simulink model "exploratory_journey"  (R2016a)
settings: Solver=FixedStepAuto  StartTime=0.0  StopTime=Param.T  FixedStep=Param.deltaT  RelTol=1e-3
undefined symbols (not defined in the file or in its folder): drawExpPath, Param, updateExpPosn, X, Y, Z
libraries: robotlib x6
settings Model: Creator=Emily  LastModifiedBy=Emily

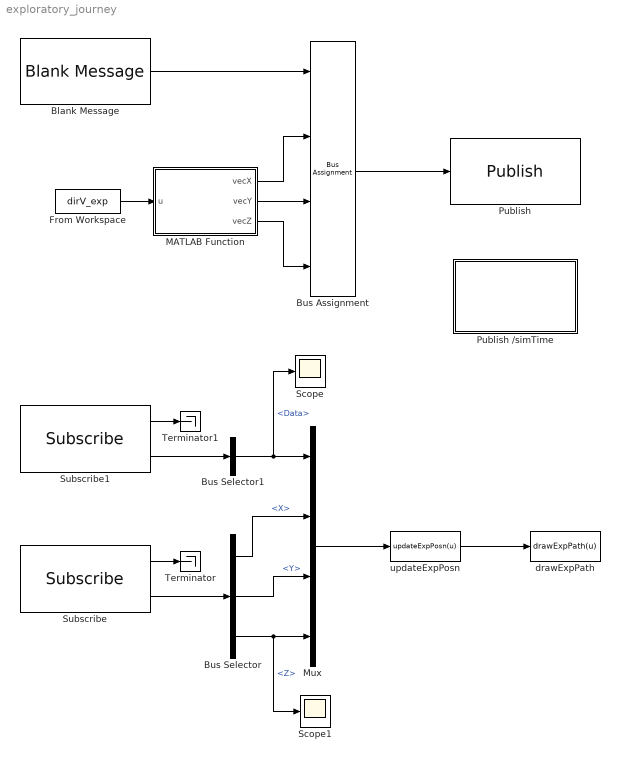
== system exploratory_journey ==
  Blank Message : robotlib/Blank Message  SourceLibraryInfo=This block requires Robotics System Toolbox  messageType=geometry_msgs/Vector3  SampleTime=inf
  Bus Assignment : BusAssignment  AssignedSignals=X,Y,Z
  Bus Selector : BusSelector  OutputSignals=X,Y,Z
  Bus Selector1 : BusSelector  OutputSignals=Data
  From Workspace : FromWorkspace  VariableName=dirV_exp  SampleTime=Param.deltaT  OutputAfterFinalValue=Holding final value
  MATLAB Function : MATLAB Function  TreatAsAtomicUnit=on
  Mux : Mux  Inputs=[1 1 1 1]
  Publish : robotlib/Publish  SourceLibraryInfo=This block requires Robotics System Toolbox  topicSource=Specify your own  topic=/simDir  messageType=geometry_msgs/Vector3  messageQueueLength=1
  Publish /simTime : Subsystem
  Scope : Scope
  Scope1 : Scope
  Subscribe : robotlib/Subscribe  SourceLibraryInfo=This block requires Robotics System Toolbox  topicSource=Specify your own  topic=/simDir  messageType=geometry_msgs/Vector3  sampleTime=-1  messageQueueLength=1
  Subscribe1 : robotlib/Subscribe  SourceLibraryInfo=This block requires Robotics System Toolbox  topicSource=Specify your own  topic=/simTime  messageType=std_msgs/Float64  sampleTime=-1  messageQueueLength=1
  Terminator : Terminator
  Terminator1 : Terminator
  drawExpPath : MATLABFcn  MATLABFcn=drawExpPath(u)  OutputDimensions=0
  updateExpPosn : MATLABFcn  MATLABFcn=updateExpPosn(u)  OutputDimensions=4
  wires:
  Blank Message/1 -> Bus Assignment/1
  Bus Assignment/1 -> Publish/1
  Subscribe/1 -> Terminator/1
  Subscribe/2 -> Bus Selector/1
  Subscribe1/1 -> Terminator1/1
  Subscribe1/2 -> Bus Selector1/1
  Mux/1 -> updateExpPosn/1
  updateExpPosn/1 -> drawExpPath/1
  Bus Selector1/1 -> Scope/1, Mux/1  "<Data>"
  Bus Selector/1 -> Mux/2  "<X>"
  Bus Selector/2 -> Mux/3  "<Y>"
  Bus Selector/3 -> Scope1/1, Mux/4  "<Z>"
  From Workspace/1 -> MATLAB Function/1(u)
  MATLAB Function/2(vecY) -> Bus Assignment/3
  MATLAB Function/1(vecX) -> Bus Assignment/2
  MATLAB Function/3(vecZ) -> Bus Assignment/4

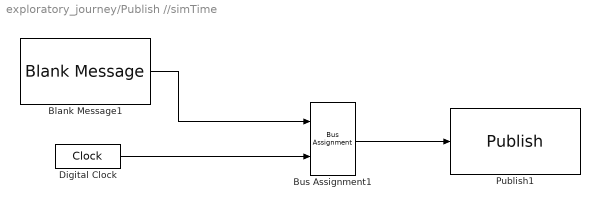
== system exploratory_journey/Publish //simTime ==
  Blank Message1 : robotlib/Blank Message  SourceLibraryInfo=This block requires Robotics System Toolbox  messageType=std_msgs/Float64  SampleTime=inf
  Bus Assignment1 : BusAssignment  AssignedSignals=Data
  Digital Clock : DigitalClock  SampleTime=Param.deltaT
  Publish1 : robotlib/Publish  SourceLibraryInfo=This block requires Robotics System Toolbox  topicSource=Specify your own  topic=/simTime  messageType=std_msgs/Float64  messageQueueLength=1
  wires:
  Digital Clock/1 -> Bus Assignment1/2
  Bus Assignment1/1 -> Publish1/1
  Blank Message1/1 -> Bus Assignment1/1

== matlab function exploratory_journey/MATLAB Function ==
  data: u input; vecX output; vecY output; vecZ output
% returns the individual elements of the dirV_exp vector
% inputs:
%   u, a 1x3 vector (row of dirV_exp)
%   time (dirV_exp(:,1)) is used as sample time, not passed to function
% outputs:
%   vecX, the x element of dirV_exp
%   vecY, the y element of dirV_exp
%   vecZ, the z element of dirV_exp

function [vecX,vecY,vecZ] = dirVecs(u)

    vecX = u(1);
    vecY = u(2);
    vecZ = u(3);
    
end
